simulink model "gNautilusDemo3"  (R2017a)
settings: Solver=FixedStepDiscrete  StartTime=0.0  StopTime=6000.0  RelTol=1e-3  EnableMultiTasking=on
model workspace (MAT data in the model file):
  cfg_native : struct (value not decoded)
  en_add_channels = 127
  host_ip = 2130706433
  host_port = 50223
  local_ip = 2130706433
  local_port = 50224
  num_en_channels = 32
  num_samples = 8
  sample_rate = 250
  serial_number = 'NR-2018.09.02'
undefined symbols (not defined in the file or in its folder): NR
libraries: gtecHighspeedLib x8, gNautilusLib x1, gNautilusTools x1
settings Model: ModifiedByFormat=g.tec  Creator=g.tec medical engineering  LastModifiedBy=g.tec
settings DataIOCC: LimitDataPoints=on  SaveFormat=Array  SignalLoggingSaveFormat=ModelDataLogs
settings OptimizationCC: ExpressionDepthLimit=2147483647  InitFltsAndDblsToZero=on  LifeSpan=inf
settings DebuggingCC: UnderspecifiedInitializationDetection=Classic  MergeDetectMultiDrivingBlocksExec=none  SolverPrmCheckMsg=warning  FcnCallInpInsideContextMsg=warning  FrameProcessingCompatibilityMsg=none  StateNameClashWarn=warning  SFUnexpectedBacktrackingDiag=warning  SFNoUnconditionalDefaultTransitionDiag=warning  SFExecutionAtInitializationDiag=none
settings HardwareCC: ProdBitPerPointer=32  ProdBitPerSizeT=32  ProdBitPerPtrDiffT=32  ProdLargestAtomicFloat=None  ProdIntDivRoundTo=Undefined  ProdEndianess=Unspecified  ProdWordSize=32  ProdHWDeviceType=32-bit Generic
settings ModelReferenceCC: PropagateSignalLabelsOutOfModel=off
settings GRTTargetCC: TargetLangStandard=C89/C90 (ANSI)  GeneratePreprocessorConditionals=Disable all  CombineOutputUpdateFcns=off  GRTInterface=on
settings ConfigComp: CovMetricSettings=dw  CovHtmlReporting=on  CovSaveCumulativeToWorkspaceVar=on  CovSaveSingleToWorkspaceVar=on  CovExternalEMLEnable=off

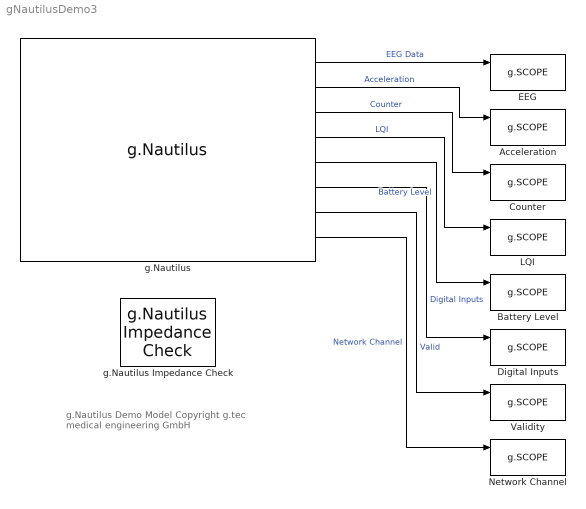
== system gNautilusDemo3 ==
  note: g.Nautilus Demo Model
      | Copyright g.tec medical engineering GmbH
  Acceleration : gtecHighspeedLib/g.SCOPE
      settings: SourceProductName=g.tec Highspeed Library
  Battery Level : gtecHighspeedLib/g.SCOPE
      settings: SourceProductName=g.tec Highspeed Library
  Counter : gtecHighspeedLib/g.SCOPE
      settings: SourceProductName=g.tec Highspeed Library
  Digital Inputs : gtecHighspeedLib/g.SCOPE
      settings: SourceProductName=g.tec Highspeed Library
  EEG : gtecHighspeedLib/g.SCOPE
      settings: SourceProductName=g.tec Highspeed Library
  LQI : gtecHighspeedLib/g.SCOPE
      settings: SourceProductName=g.tec Highspeed Library
  Network Channel : gtecHighspeedLib/g.SCOPE
      settings: SourceProductName=g.tec Highspeed Library
  Validity : gtecHighspeedLib/g.SCOPE
      settings: SourceProductName=g.tec Highspeed Library
  g.Nautilus : gNautilusLib/g.Nautilus  Tag=g.Nautilus  Description=Operates a g.Nautilus device and provides acquired data on its outputs.  sample_rate=250  local_ip=2130706433  local_port=50224  host_ip=2130706433  host_port=50223  serial_number=NR-2018.09.02  num_samples=8  num_en_channels=32  add_channels=127
      settings: SourceProductName=g.Nautilus
  g.Nautilus Impedance Check : gNautilusTools/g.Nautilus Impedance Check
  wires:
  g.Nautilus/2 -> Acceleration/1  "Acceleration"
  g.Nautilus/3 -> Counter/1  "Counter"
  g.Nautilus/4 -> LQI/1  "LQI"
  g.Nautilus/5 -> Battery Level/1  "Battery Level"
  g.Nautilus/6 -> Digital Inputs/1  "Digital Inputs"
  g.Nautilus/7 -> Validity/1  "Valid"
  g.Nautilus/8 -> Network Channel/1  "Network Channel"
  g.Nautilus/1 -> EEG/1  "EEG Data"
